simulink model "eyemodel"  (R2019a)
settings: Solver=VariableStepAuto  StartTime=constant*(i-1)/(velocity/fps)  StopTime=3  RelTol=1e-3
values from neighbouring files (symbols this model uses):
  B = 0.018    [Code.m]
  J = 4.3 * 10e-5    (= 0.00043)    [Code.m]
  K = 0.86    [Code.m]
  Kse = 1.8    [Code.m]
  N_AG_Pulse = PH    [Code.m]
  N_AG_Step = step1 + 0.8*(dTheta)    [Code.m]
  N_AN_Pulse = 0.5 + pulse1*exp((-dTheta)/2.5)    [Code.m]
  N_AN_Step = step2-0.06*(dTheta)    [Code.m]
  PW = 40e-3    (= 0.04)    [Code.m]
  r = pi/180    (= 0.0174532925199)    [Code.m]
  TauAG_AC = (13-0.1*(dTheta))*1e-3    [Code.m]
  zero = 10e-3    (= 0.01)    [Code.m]
settings Model: Creator=Mert Beser  LastModifiedBy=Mert Beser

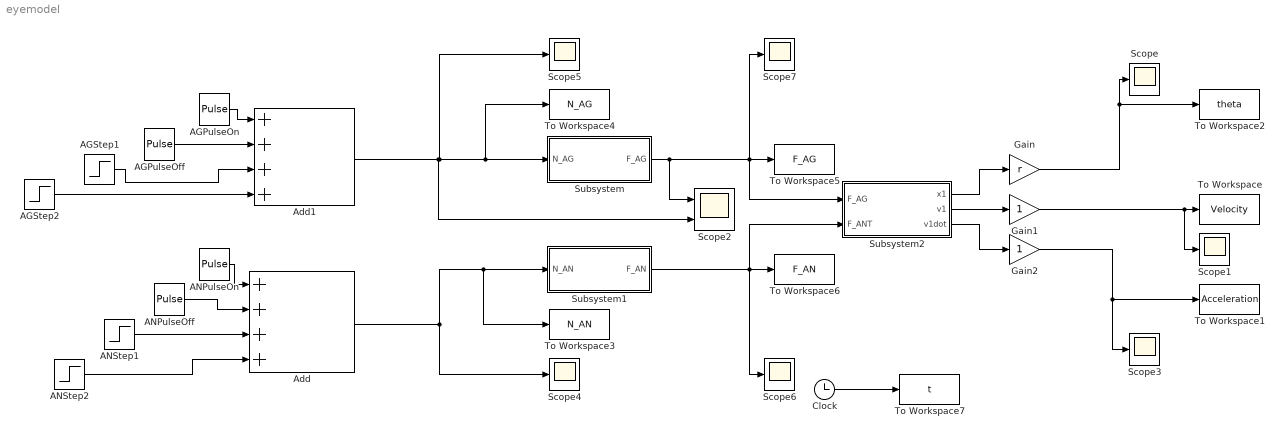
== system eyemodel ==
  AGPulseOff : DiscretePulseGenerator  PulseType=Time based  Amplitude=-N_AG_Pulse  Period=2*PW  PulseWidth=50  PhaseDelay=zero+2*PW
  AGPulseOn : DiscretePulseGenerator  PulseType=Time based  Amplitude=N_AG_Pulse  Period=2*PW  PulseWidth=50  PhaseDelay=zero
  AGStep1 : Step  Time=zero+PW  After=N_AG_Step  SampleTime=0
  AGStep2 : Step  Time=zero  Before=16  After=0  SampleTime=0
  ANPulseOff : DiscretePulseGenerator  PulseType=Time based  Amplitude=-N_AN_Pulse  Period=2*PW  PulseWidth=65  PhaseDelay=zero+2*PW-0.003
  ANPulseOn : DiscretePulseGenerator  PulseType=Time based  Amplitude=N_AN_Pulse  Period=2*PW  PulseWidth=65  PhaseDelay=zero-0.003
  ANStep1 : Step  Time=zero+PW+0.003  After=N_AN_Step  SampleTime=0
  ANStep2 : Step  Time=zero-0.003  Before=16  After=0  SampleTime=0
  Add : Sum  Inputs=++++
  Add1 : Sum  Inputs=++++
  Clock : Clock
  Gain : Gain  Gain=r
  Gain1 : Gain
  Gain2 : Gain
  Scope{,1,3..7} (7 alike) : Scope
  Scope2 : Scope  NumInputPorts=2
  Subsystem : Subsystem
  Subsystem1 : Subsystem
  Subsystem2 : Subsystem
  To Workspace : ToWorkspace  VariableName=Velocity  SaveFormat=Timeseries  SampleTime=-1
  To Workspace1 : ToWorkspace  VariableName=Acceleration  SaveFormat=Timeseries  SampleTime=-1
  To Workspace2 : ToWorkspace  VariableName=theta  SampleTime=-1
  To Workspace3 : ToWorkspace  VariableName=N_AN  SaveFormat=Timeseries  SampleTime=-1
  To Workspace4 : ToWorkspace  VariableName=N_AG  SaveFormat=Timeseries  SampleTime=-1
  To Workspace5 : ToWorkspace  VariableName=F_AG  SaveFormat=Timeseries  SampleTime=-1
  To Workspace6 : ToWorkspace  VariableName=F_AN  SaveFormat=Timeseries  SampleTime=-1
  To Workspace7 : ToWorkspace  VariableName=t  SampleTime=-1
  wires:
  Subsystem/1(F_AG) -> Scope2/1, Scope7/1, To Workspace5/1, Subsystem2/1(F_AG)
  Subsystem1/1(F_AN) -> Scope6/1, To Workspace6/1, Subsystem2/2(F_ANT)
  Subsystem2/3(v1dot) -> Gain2/1
  Subsystem2/2(v1) -> Gain1/1
  Subsystem2/1("x1 ") -> Gain/1
  Gain1/1 -> Scope1/1, To Workspace/1
  Gain2/1 -> Scope3/1, To Workspace1/1
  Gain/1 -> Scope/1, To Workspace2/1
  Add1/1 -> Scope2/2, Scope5/1, To Workspace4/1, Subsystem/1(N_AG)
  Add/1 -> To Workspace3/1, Subsystem1/1(N_AN), Scope4/1
  ANStep2/1 -> Add/4
  AGStep2/1 -> Add1/4
  ANPulseOn/1 -> Add/1
  ANStep1/1 -> Add/3
  AGStep1/1 -> Add1/3
  AGPulseOn/1 -> Add1/1
  ANPulseOff/1 -> Add/2
  AGPulseOff/1 -> Add1/2
  Clock/1 -> To Workspace7/1

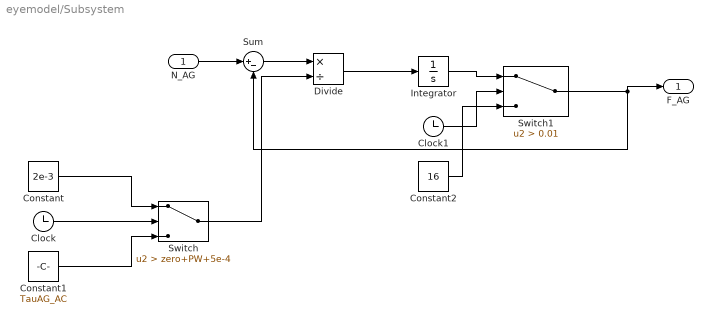
== system eyemodel/Subsystem ==
  N_AG : Inport
  Clock : Clock
  Clock1 : Clock
  Constant : Constant  Value=2e-3
  Constant1 : Constant  Value=TauAG_AC
  Constant2 : Constant  Value=16
  Divide : Product  Inputs=*/
  Integrator : Integrator
  Sum : Sum  Inputs=|+-
  Switch : Switch  Criteria=u2 > Threshold  Threshold=zero+PW+5e-4
  Switch1 : Switch  Criteria=u2 > Threshold  Threshold=0.01
  F_AG : Outport
  wires:
  Divide/1 -> Integrator/1
  Constant1/1 -> Switch/3
  Clock/1 -> Switch/2
  Constant2/1 -> Switch1/3
  Switch1/1 -> F_AG/1, Sum/2
  Clock1/1 -> Switch1/2
  Integrator/1 -> Switch1/1
  Switch/1 -> Divide/2
  Sum/1 -> Divide/1
  N_AG/1 -> Sum/1
  Constant/1 -> Switch/1

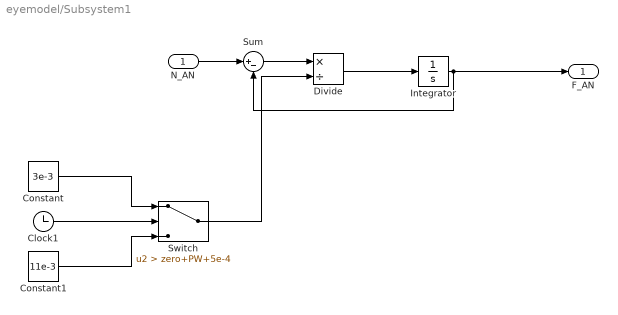
== system eyemodel/Subsystem1 ==
  N_AN : Inport
  Clock1 : Clock
  Constant : Constant  Value=3e-3
  Constant1 : Constant  Value=11e-3
  Divide : Product  Inputs=*/
  Integrator : Integrator
  Sum : Sum  Inputs=|+-
  Switch : Switch  Criteria=u2 > Threshold  Threshold=zero+PW+5e-4
  F_AN : Outport
  wires:
  Switch/1 -> Divide/2
  N_AN/1 -> Sum/1
  Constant/1 -> Switch/1
  Constant1/1 -> Switch/3
  Clock1/1 -> Switch/2
  Divide/1 -> Integrator/1
  Sum/1 -> Divide/1
  Integrator/1 -> Sum/2, F_AN/1

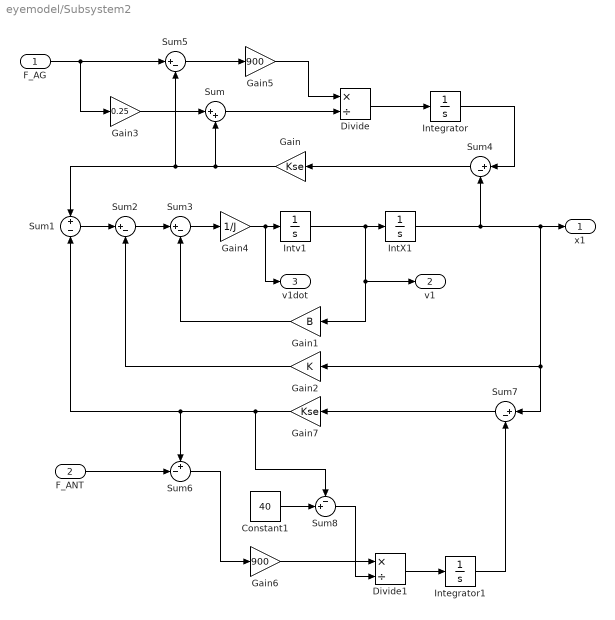
== system eyemodel/Subsystem2 ==
  F_AG : Inport
  F_ANT : Inport  Port=2
  Constant1 : Constant  Value=40
  Divide : Product  Inputs=*/
  Divide1 : Product  Inputs=*/
  Gain : Gain  Gain=Kse
  Gain1 : Gain  Gain=B
  Gain2 : Gain  Gain=K
  Gain3 : Gain  Gain=0.25
  Gain4 : Gain  Gain=1/J
  Gain5 : Gain  Gain=900
  Gain6 : Gain  Gain=900
  Gain7 : Gain  Gain=Kse
  IntX1 : Integrator
  Integrator : Integrator
  Integrator1 : Integrator
  Intv1 : Integrator
  Sum : Sum  Inputs=|++
  Sum1 : Sum  Inputs=+|-
  Sum{2..5,7} (5 alike) : Sum  Inputs=|+-
  Sum6 : Sum  Inputs=+-|
  Sum8 : Sum  Inputs=-+|
  "x1 " : Outport
  v1 : Outport  Port=2
  v1dot : Outport  Port=3
  wires:
  Integrator/1 -> Sum4/1
  F_AG/1 -> Sum5/1, Gain3/1
  Sum5/1 -> Gain5/1
  Sum7/1 -> Gain7/1
  Gain5/1 -> Divide/1
  Sum1/1 -> Sum2/1
  Sum3/1 -> Gain4/1
  Constant1/1 -> Sum8/2
  Gain2/1 -> Sum2/2
  IntX1/1 -> Sum7/1, Gain2/1, "x1 "/1, Sum4/2
  Gain1/1 -> Sum3/2
  Sum4/1 -> Gain/1
  Sum/1 -> Divide/2
  Gain4/1 -> v1dot/1, Intv1/1
  Gain3/1 -> Sum/1
  F_ANT/1 -> Sum6/2
  Sum2/1 -> Sum3/1
  Sum8/1 -> Divide1/2
  Divide/1 -> Integrator/1
  Intv1/1 -> Gain1/1, v1/1, IntX1/1
  Sum6/1 -> Gain6/1
  Gain/1 -> Sum/2, Sum5/2, Sum1/1
  Gain7/1 -> Sum6/1, Sum1/2, Sum8/1
  Integrator1/1 -> Sum7/2
  Divide1/1 -> Integrator1/1
  Gain6/1 -> Divide1/1
